simulink model "NeuroControl_Loudspeaker_offline"  (R2016a)
settings: Solver=ode5  StartTime=0.0  StopTime=SimTime  FixedStep=1/fsSim  RelTol=1e-3
values from neighbouring files (symbols this model uses):
  AaLinear = [0,1,0,0; -(K)/Md,-Rmd/Md,0,A/Md; 0,0,0,1; 0,-A/(L0+Ld),-(1/Cd)/(L0+Ld),-(Re0+Red)/(L0+Ld)]    [NeuroControl_loudspeaker.m]    (also in NeuroControl_loudspeaker2.m; NeuroControl_loudspeaker_LinearPlusNN.m; NeuroControl_loudspeaker_MoreLikeMachineLearning.m; NeuroControl_loudspeaker_MoreLikeMachineLearning_deep.m)
  Anlr = zeros(4,4)    [NeuroControl_loudspeaker.m]    (also in NeuroControl_loudspeaker2.m; NeuroControl_loudspeaker_LinearPlusNN.m; NeuroControl_loudspeaker_MoreLikeMachineLearning.m; NeuroControl_loudspeaker_MoreLikeMachineLearning_deep.m)
  Anlr2 = zeros(4,4)    [NeuroControl_loudspeaker.m]    (also in NeuroControl_loudspeaker2.m; NeuroControl_loudspeaker_LinearPlusNN.m; NeuroControl_loudspeaker_MoreLikeMachineLearning.m; NeuroControl_loudspeaker_MoreLikeMachineLearning_deep.m)
  Anlr3 = zeros(4,4)    [NeuroControl_loudspeaker.m]    (also in NeuroControl_loudspeaker2.m; NeuroControl_loudspeaker_LinearPlusNN.m; NeuroControl_loudspeaker_MoreLikeMachineLearning.m; NeuroControl_loudspeaker_MoreLikeMachineLearning_deep.m)
  Atemp = A    (= 5.62)    [NeuroControl_loudspeaker.m]    (also in NeuroControl_loudspeaker2.m; NeuroControl_loudspeaker_LinearPlusNN.m; NeuroControl_loudspeaker_MoreLikeMachineLearning.m; NeuroControl_loudspeaker_MoreLikeMachineLearning_deep.m)
  Ba = [0,0,0,1/(L0+Ld)]'    [NeuroControl_loudspeaker.m]    (also in NeuroControl_loudspeaker2.m; NeuroControl_loudspeaker_LinearPlusNN.m; NeuroControl_loudspeaker_MoreLikeMachineLearning.m; NeuroControl_loudspeaker_MoreLikeMachineLearning_deep.m)
  Fb = FbSVD    [NeuroControl_loudspeaker.m]    (also in NeuroControl_loudspeaker2.m; NeuroControl_loudspeaker_LinearPlusNN.m; NeuroControl_loudspeaker_MoreLikeMachineLearning.m = Y3; NeuroControl_loudspeaker_MoreLikeMachineLearning_deep.m = Fbtemp)
  fInput = 60    [NeuroControl_loudspeaker.m]    (also in NeuroControl_loudspeaker2.m; NeuroControl_loudspeaker_LinearPlusNN.m; NeuroControl_loudspeaker_MoreLikeMachineLearning.m; NeuroControl_loudspeaker_MoreLikeMachineLearning_deep.m)
  fs = fs/downrate    (= 48000)    [NeuroControl_loudspeaker.m]    (also in NeuroControl_loudspeaker2.m; NeuroControl_loudspeaker_LinearPlusNN.m; NeuroControl_loudspeaker_MoreLikeMachineLearning.m; NeuroControl_loudspeaker_MoreLikeMachineLearning_deep.m)
  fsSim = 48000    [NeuroControl_loudspeaker.m]    (also in NeuroControl_loudspeaker2.m; NeuroControl_loudspeaker_LinearPlusNN.m; NeuroControl_loudspeaker_MoreLikeMachineLearning.m; NeuroControl_loudspeaker_MoreLikeMachineLearning_deep.m)
  G = Gt'    [NeuroControl_loudspeaker.m]    (also in NeuroControl_loudspeaker2.m; NeuroControl_loudspeaker_LinearPlusNN.m; NeuroControl_loudspeaker_MoreLikeMachineLearning.m; NeuroControl_loudspeaker_MoreLikeMachineLearning_deep.m)
  gain = 1/zpkerasys(1,1).k    [NeuroControl_loudspeaker.m]    (also in NeuroControl_loudspeaker2.m; NeuroControl_loudspeaker_LinearPlusNN.m; NeuroControl_loudspeaker_MoreLikeMachineLearning.m; NeuroControl_loudspeaker_MoreLikeMachineLearning_deep.m)
  InputGain = 1    [NeuroControl_loudspeaker.m]    (also in NeuroControl_loudspeaker2.m; NeuroControl_loudspeaker_LinearPlusNN.m; NeuroControl_loudspeaker_MoreLikeMachineLearning.m; NeuroControl_loudspeaker_MoreLikeMachineLearning_deep.m)
  inputGainForPushingNonlinearity = 5    [NeuroControl_loudspeaker.m]    (also in NeuroControl_loudspeaker2.m; NeuroControl_loudspeaker_LinearPlusNN.m = 10; NeuroControl_loudspeaker_MoreLikeMachineLearning.m = 10; NeuroControl_loudspeaker_MoreLikeMachineLearning_deep.m = 10)
  inverseFilterGainCompensation = 1/0.0054    (= 185.185185185)    [NeuroControl_loudspeaker.m]    (also in NeuroControl_loudspeaker2.m; NeuroControl_loudspeaker_LinearPlusNN.m; NeuroControl_loudspeaker_MoreLikeMachineLearning.m; NeuroControl_loudspeaker_MoreLikeMachineLearning_deep.m)
  K = Kd    (= 4538)    [NeuroControl_loudspeaker.m]    (also in NeuroControl_loudspeaker2.m; NeuroControl_loudspeaker_LinearPlusNN.m; NeuroControl_loudspeaker_MoreLikeMachineLearning.m; NeuroControl_loudspeaker_MoreLikeMachineLearning_deep.m)
  noise = 0    [NeuroControl_loudspeaker.m]    (also in NeuroControl_loudspeaker2.m; NeuroControl_loudspeaker_LinearPlusNN.m; NeuroControl_loudspeaker_MoreLikeMachineLearning.m; NeuroControl_loudspeaker_MoreLikeMachineLearning_deep.m)
  ObserverNorm = 1    [NeuroControl_loudspeaker.m]    (also in NeuroControl_loudspeaker2.m; NeuroControl_loudspeaker_LinearPlusNN.m; NeuroControl_loudspeaker_MoreLikeMachineLearning.m; NeuroControl_loudspeaker_MoreLikeMachineLearning_deep.m)
  plantInputGainCompensationFb = 1/1.15    (= 0.869565217391)    [NeuroControl_loudspeaker.m]    (also in NeuroControl_loudspeaker2.m; NeuroControl_loudspeaker_LinearPlusNN.m; NeuroControl_loudspeaker_MoreLikeMachineLearning.m; NeuroControl_loudspeaker_MoreLikeMachineLearning_deep.m)
  pole = z_svd    [NeuroControl_loudspeaker.m]    (also in NeuroControl_loudspeaker2.m; NeuroControl_loudspeaker_LinearPlusNN.m; NeuroControl_loudspeaker_MoreLikeMachineLearning.m; NeuroControl_loudspeaker_MoreLikeMachineLearning_deep.m)
  Rmd = 2.34    [NeuroControl_loudspeaker.m]    (also in NeuroControl_loudspeaker2.m; NeuroControl_loudspeaker_LinearPlusNN.m; NeuroControl_loudspeaker_MoreLikeMachineLearning.m; NeuroControl_loudspeaker_MoreLikeMachineLearning_deep.m)
  SignalChange = temp    (= 0)    [NeuroControl_loudspeaker.m]    (also in NeuroControl_loudspeaker2.m; NeuroControl_loudspeaker_LinearPlusNN.m; NeuroControl_loudspeaker_MoreLikeMachineLearning.m; NeuroControl_loudspeaker_MoreLikeMachineLearning_deep.m)
  sys_era_c = d2c(sys_era,'zoh')    [NeuroControl_loudspeaker.m]    (also in NeuroControl_loudspeaker2.m; NeuroControl_loudspeaker_LinearPlusNN.m; NeuroControl_loudspeaker_MoreLikeMachineLearning.m; NeuroControl_loudspeaker_MoreLikeMachineLearning_deep.m)
  zero = zpkerasys(1,1).p{1,1}    [NeuroControl_loudspeaker.m]    (also in NeuroControl_loudspeaker2.m; NeuroControl_loudspeaker_LinearPlusNN.m; NeuroControl_loudspeaker_MoreLikeMachineLearning.m; NeuroControl_loudspeaker_MoreLikeMachineLearning_deep.m)
undefined symbols (not defined in the file or in its folder): a, b
libraries: simulink x1
settings Model: Creator=kadowaki  LastModifiedBy=kadowaki
settings DataIOCC: LimitDataPoints=on  SaveFormat=Array  SignalLoggingSaveFormat=ModelDataLogs  SignalLogging=off
settings OptimizationCC: ExpressionDepthLimit=2147483647  InitFltsAndDblsToZero=on
settings DebuggingCC: UnderspecifiedInitializationDetection=Classic  MergeDetectMultiDrivingBlocksExec=none  SolverPrmCheckMsg=warning  FcnCallInpInsideContextMsg=UseLocalSettings  StateNameClashWarn=warning
settings HardwareCC: ProdBitPerPointer=32  ProdLargestAtomicFloat=None  ProdIntDivRoundTo=Undefined  ProdEndianess=Unspecified  ProdWordSize=32  ProdHWDeviceType=32-bit Generic
settings ModelReferenceCC: ModelReferenceMinAlgLoopOccurrences=on  PropagateSignalLabelsOutOfModel=off
settings GRTTargetCC: GeneratePreprocessorConditionals=Use local settings  CombineOutputUpdateFcns=off  GRTInterface=on
settings ConfigComp: CovModelRefEnable=Off

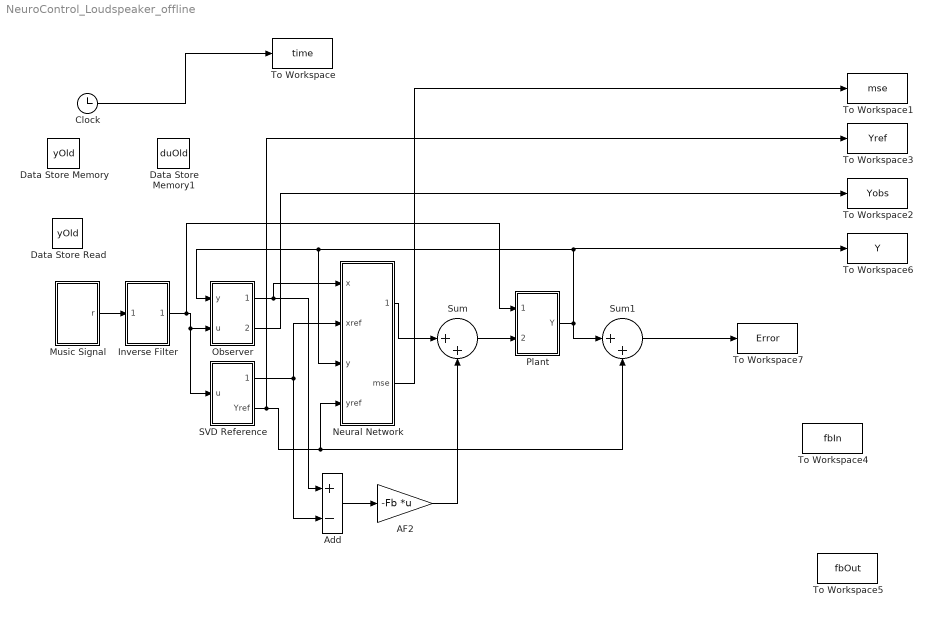
== system NeuroControl_Loudspeaker_offline ==
  AF2 : Gain  Gain=-Fb  Multiplication=Matrix(K*u)
  Add : Sum  Inputs=+-
  Clock : Clock
  Data Store Memory : DataStoreMemory  DataStoreName=yOld  ReadBeforeWriteMsg=warning  WriteAfterWriteMsg=warning  WriteAfterReadMsg=warning  ShowAdditionalParam=off  OutDataTypeStr=double
  Data Store Memory1 : DataStoreMemory  DataStoreName=duOld  ReadBeforeWriteMsg=warning  WriteAfterWriteMsg=warning  WriteAfterReadMsg=warning  ShowAdditionalParam=off  OutDataTypeStr=double
  Data Store Read : DataStoreRead  DataStoreName=yOld
  Inverse Filter : Subsystem
  Music Signal : Subsystem
  Neural Network : MATLAB Function  TreatAsAtomicUnit=on
      settings: MinAlgLoopOccurrences=on
  Observer : Subsystem
  Plant : Subsystem
  SVD Reference : Subsystem
  Sum : Sum  Inputs=|++
  Sum1 : Sum  Inputs=|++
  To Workspace : ToWorkspace  VariableName=time  SampleTime=-1
  To Workspace1 : ToWorkspace  VariableName=mse  SampleTime=-1
  To Workspace2 : ToWorkspace  VariableName=Yobs  SampleTime=-1
  To Workspace3 : ToWorkspace  VariableName=Yref  SampleTime=-1
  To Workspace4 : ToWorkspace  VariableName=fbIn  SampleTime=-1
  To Workspace5 : ToWorkspace  VariableName=fbOut  SampleTime=-1
  To Workspace6 : ToWorkspace  VariableName=Y  SampleTime=-1
  To Workspace7 : ToWorkspace  VariableName=Error  SampleTime=-1
  wires:
  Clock/1 -> To Workspace/1
  Neural Network/1(duOut) -> Sum/1
  Sum/1 -> Plant/2(control)
  Plant/1(Y) -> Sum1/1, Neural Network/3(y), Observer/1(y), To Workspace6/1
  Inverse Filter/1(Out1) -> Plant/1(music), SVD Reference/1(u), Observer/2(u)
  SVD Reference/1(Xref) -> Add/2, Neural Network/2(xref)
  Observer/1(xBar) -> Add/1, Neural Network/1(x)
  Music Signal/1(r) -> Inverse Filter/1(In1)
  SVD Reference/2(Yref) -> Neural Network/4(yref), Sum1/2, To Workspace3/1
  Sum1/1 -> To Workspace7/1
  Add/1 -> AF2/1
  AF2/1 -> Sum/2
  Observer/2(ybar) -> To Workspace2/1
  Neural Network/2(mse) -> To Workspace1/1

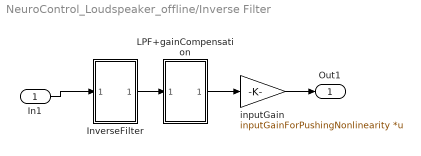
== system NeuroControl_Loudspeaker_offline/Inverse Filter ==
  In1 : Inport
  InverseFilter : Subsystem
  LPF+gainCompensation : Subsystem
  inputGain : Gain  Gain=inputGainForPushingNonlinearity  Multiplication=Matrix(K*u)
  Out1 : Outport
  wires:
  In1/1 -> InverseFilter/1(In1)
  InverseFilter/1(Out1) -> LPF+gainCompensation/1(In1)
  LPF+gainCompensation/1(Out1) -> inputGain/1
  inputGain/1 -> Out1/1

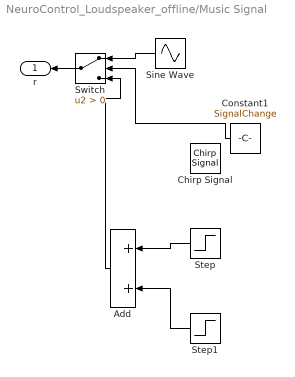
== system NeuroControl_Loudspeaker_offline/Music Signal ==
  Add : Sum
  Chirp Signal : simulink/Sources/Chirp Signal  f1=0.1  T=2  f2=fs/2
  Constant1 : Constant  Value=SignalChange
  Sine Wave : Sin  Amplitude=InputGain  Frequency=2*pi*fInput  SampleTime=0
  Step : Step  Time=0  After=InputGain  SampleTime=0
  Step1 : Step  Time=1/fsSim  After=-InputGain  SampleTime=0
  Switch : Switch  Criteria=u2 > Threshold
  r : Outport
  wires:
  Switch/1 -> r/1
  Constant1/1 -> Switch/2
  Sine Wave/1 -> Switch/1
  Step/1 -> Add/1
  Step1/1 -> Add/2
  Add/1 -> Switch/3

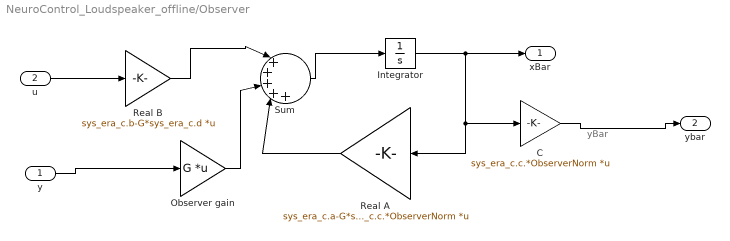
== system NeuroControl_Loudspeaker_offline/Observer ==
  note: yBar
  y : Inport
  u : Inport  Port=2
  C : Gain  Gain=sys_era_c.c.*ObserverNorm  Multiplication=Matrix(K*u)
  Integrator : Integrator
  Observer gain : Gain  Gain=G  Multiplication=Matrix(K*u)
  Real A : Gain  Gain=sys_era_c.a-G*sys_era_c.c.*ObserverNorm  Multiplication=Matrix(K*u)
  Real B : Gain  Gain=sys_era_c.b-G*sys_era_c.d  Multiplication=Matrix(K*u)
  Sum : Sum  Inputs=|+++++
  xBar : Outport
  ybar : Outport  Port=2
  wires:
  Sum/1 -> Integrator/1
  Integrator/1 -> Real A/1, C/1, xBar/1
  Real A/1 -> Sum/4
  u/1 -> Real B/1
  Real B/1 -> Sum/1
  y/1 -> Observer gain/1
  C/1 -> ybar/1
  Observer gain/1 -> Sum/3

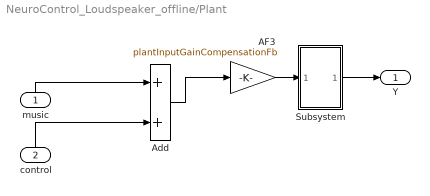
== system NeuroControl_Loudspeaker_offline/Plant ==
  music : Inport
  control : Inport  Port=2
  AF3 : Gain  Gain=plantInputGainCompensationFb
  Add : Sum
  Subsystem : Subsystem  TreatAsAtomicUnit=on
      settings: MinAlgLoopOccurrences=on
  Y : Outport
  wires:
  Subsystem/1(Out1) -> Y/1
  AF3/1 -> Subsystem/1(In2)
  music/1 -> Add/1
  control/1 -> Add/2
  Add/1 -> AF3/1

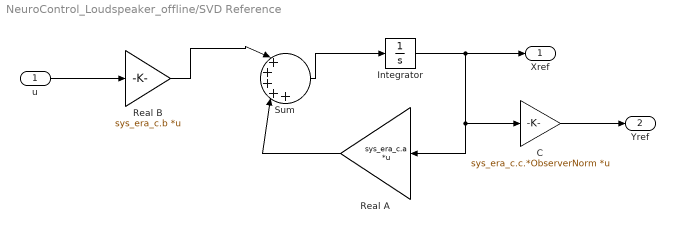
== system NeuroControl_Loudspeaker_offline/SVD Reference ==
  u : Inport
  C : Gain  Gain=sys_era_c.c.*ObserverNorm  Multiplication=Matrix(K*u)
  Integrator : Integrator
  Real A : Gain  Gain=sys_era_c.a  Multiplication=Matrix(K*u)
  Real B : Gain  Gain=sys_era_c.b  Multiplication=Matrix(K*u)
  Sum : Sum  Inputs=|+++++
  Xref : Outport
  Yref : Outport  Port=2
  wires:
  Sum/1 -> Integrator/1
  Integrator/1 -> Real A/1, C/1, Xref/1
  Real A/1 -> Sum/4
  u/1 -> Real B/1
  Real B/1 -> Sum/1
  C/1 -> Yref/1

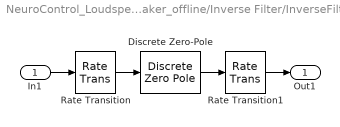
== system NeuroControl_Loudspeaker_offline/Inverse Filter/InverseFilter ==
  In1 : Inport
  Discrete Zero-Pole : DiscreteZeroPole  Zeros=zero  Poles=pole  Gain=gain  SampleTime=1/fs
  Rate Transition : RateTransition
  Rate Transition1 : RateTransition
  Out1 : Outport
  wires:
  Rate Transition/1 -> Discrete Zero-Pole/1
  Discrete Zero-Pole/1 -> Rate Transition1/1
  In1/1 -> Rate Transition/1
  Rate Transition1/1 -> Out1/1

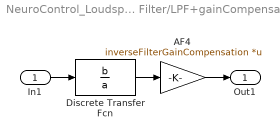
== system NeuroControl_Loudspeaker_offline/Inverse Filter/LPF+gainCompensation ==
  In1 : Inport
  AF4 : Gain  Gain=inverseFilterGainCompensation  Multiplication=Matrix(K*u)
  Discrete Transfer Fcn : DiscreteTransferFcn  Numerator=b  Denominator=a
  Out1 : Outport
  wires:
  Discrete Transfer Fcn/1 -> AF4/1
  AF4/1 -> Out1/1
  In1/1 -> Discrete Transfer Fcn/1

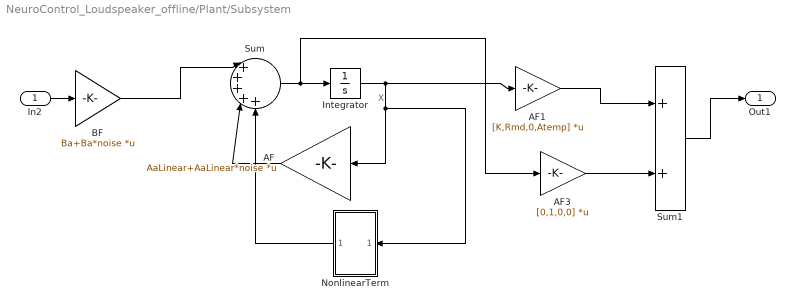
== system NeuroControl_Loudspeaker_offline/Plant/Subsystem ==
  note: X
  In2 : Inport
  AF : Gain  Gain=AaLinear+AaLinear*noise  Multiplication=Matrix(K*u)
  AF1 : Gain  Gain=[K,Rmd,0,Atemp]  Multiplication=Matrix(K*u)
  AF3 : Gain  Gain=[0,1,0,0]  Multiplication=Matrix(K*u)
  BF : Gain  Gain=Ba+Ba*noise  Multiplication=Matrix(K*u)
  Integrator : Integrator
  NonlinearTerm : Subsystem
  Sum : Sum  Inputs=|+++++
  Sum1 : Sum
  Out1 : Outport
  wires:
  BF/1 -> Sum/1
  Sum/1 -> Integrator/1, AF3/1
  Integrator/1 -> AF/1, NonlinearTerm/1(In1), AF1/1
  AF/1 -> Sum/4
  NonlinearTerm/1(Out2) -> Sum/5
  In2/1 -> BF/1
  AF1/1 -> Sum1/1
  Sum1/1 -> Out1/1
  AF3/1 -> Sum1/2

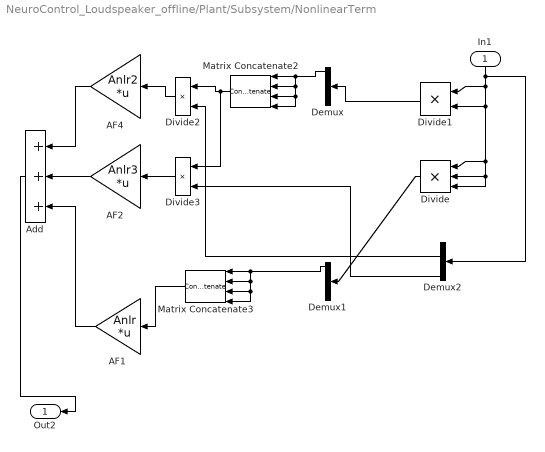
== system NeuroControl_Loudspeaker_offline/Plant/Subsystem/NonlinearTerm ==
  In1 : Inport
  AF1 : Gain  Gain=Anlr  Multiplication=Matrix(K*u)
  AF2 : Gain  Gain=Anlr3  Multiplication=Matrix(K*u)
  AF4 : Gain  Gain=Anlr2  Multiplication=Matrix(K*u)
  Add : Sum  Inputs=+++
  Demux : Demux  Outputs=[1,1,1,1]
  Demux1 : Demux  Outputs=[1,1,1,1]
  Demux2 : Demux  Outputs=[1,1,1,1]
  Divide : Product  Inputs=***
  Divide1 : Product  Inputs=**
  Divide2 : Product  Inputs=**
  Divide3 : Product  Inputs=**
  Matrix Concatenate2 : Concatenate  NumInputs=4
  Matrix Concatenate3 : Concatenate  NumInputs=4
  Out2 : Outport
  wires:
  Matrix Concatenate3/1 -> AF1/1
  Divide/1 -> Demux1/1
  In1/1 -> Demux2/1, Divide1/2, Divide/2, Divide/3, Divide/1, Divide1/1
  Demux/1 -> Matrix Concatenate2/1, Matrix Concatenate2/2, Matrix Concatenate2/3, Matrix Concatenate2/4
  Demux1/1 -> Matrix Concatenate3/1, Matrix Concatenate3/2, Matrix Concatenate3/3, Matrix Concatenate3/4
  AF2/1 -> Add/2
  AF4/1 -> Add/1
  AF1/1 -> Add/3
  Add/1 -> Out2/1
  Matrix Concatenate2/1 -> Divide2/1, Divide3/1
  Demux2/2 -> Divide2/2
  Divide2/1 -> AF4/1
  Divide3/1 -> AF2/1
  Demux2/4 -> Divide3/2
  Divide1/1 -> Demux/1

== matlab function NeuroControl_Loudspeaker_offline/Neural Network ==
  data: x input; duOut output; xref input; mse output; y input; yref input; yOld data_store_memory; duOld data_store_memory
function [duOut,mse] = fcn(x,xref,y,yref)
%% cost関数をatctual plantの出力YとYrefの差の二乗和の形に書き換える。それにともなってsigKとかも変わる
%%%%%%%%%%%%%%%%%%%%%%%%%%%%%%%%%%%%%%%%%%%%%%%%%%%%%%%%%%%%%%%%%%%%%%%%%%%%%%%%%%%%%%%%%%%%%%%%%%%%%%%%%%%%
%%

%#codegen
%配列は縦で入れる
%PRMLの5.3.2
%隠れ層はtanh,出力層は線形の活性化関数
% Input:
%   x: state vector of a plant
%   xref: reference state vector
%   h: 隠れ層のニューロン数
% Ouput:
%   du: input to compensate plant nonlinearity
%   mse: mean square error
%12input-1outputのニューラルネット
%フィードバックの機構いる？ニューラルネットだけではだめなのか。
%実装に際しては，1サンプル中にニューラルネットの計算が終わるのかという問題はある。

%過去のy保存用のグローバル変数定義
global yOld
global duOld

if isempty(yOld) == 1
    duOld = 0;
    yOld = 0;
end

%隠れ層のレイヤー数
h = 12;
%各レイヤーのユニット数
%h = [size(x,1)+1;h(:)+1;size(xref,1)];
h = [size(x,1)+1;h(:)+1;1];
%レイヤー数
L = numel(h);
W = cell(L-1);
for l = 1:L-1
    W{l} = randn(h(l),h(l+1));
end
du = cell(L);
du{1} = [1;x];
%eta = 1/size(x,2);
eta = 0.01;
maxiter = 4000;
mse = zeros(1,maxiter);
mse(1) = 1;
% %描画準備
% figure(1)
% plot(xref)
% hold on
%iteration variable
iter = 1;
%while mse(iter) > 0.0005
    iter = iter + 1;
    %forward
    %中間層出力
    l = 2;
    
    %活性化関数定義
    du{l} = tanh(W{l-1}'*du{l-1});
    
    %出力層出力
    l = 3;
    du{l} = W{l-1}'*du{l-1};
    
    %ここで一旦プラントに入力
    
    
    %ヤコビアンを求める
    deltaU = du{3} - duOld;
    deltaY = y - yOld;
    if deltaU*deltaY < 0
        jacobi = -1;
    elseif deltaU*deltaY == 0
        jacobi = 0;
    else 
        jacobi = 1;
    end
    
    %出力層ユニットに対するsigmaK
    sigK = (y - yref)*jacobi;
    %     backward
    E = y - yref;
    mse(iter) = mean(dot(E(:),E(:)));
    l = 2;
    %         df = (1-Y{l+1}.^2);
    %         dG = df.*E;
    %         dW = Y{l}*dG';
    
    sigJ = (1-du{l}.^2).*(W{l}*sigK);
    
    W{1} = W{1}-eta*(sigJ*du{1}')';
    W{2} = W{2}-eta*(sigK*du{2}')';
    
    %     if mod(iter,10) == 0
    %         figure(1)
    %         plot(Y{L})
    %     end
%     %成長の描画
%     figure(1)
%     ylim([min(xref)*1.2, max(xref)*1.2])
%     plot(du{L})
%     pause(.1)
%end
mse = mse(1:iter);
%model.W = W;
duOut = du{3};
duOld = duOut;
yOld = y;
%disp(['iteration number:',num2str(iter)])
